simulink model "ejemplo_arduino"  (R2016a)
settings: Solver=ode3  StartTime=0.0  StopTime=inf  FixedStep=0.001  RelTol=1e-3
libraries: simulink x1, sldrtlib x1, aerolibanimutils x1
settings Model: Creator=Usuario  LastModifiedBy=santd
settings DataIOCC: LimitDataPoints=on  SaveFormat=Array
settings DebuggingCC: SolverPrmCheckMsg=warning  AllowSymbolicDim=off
settings HardwareCC: ProdBitPerPointer=32  ProdLargestAtomicFloat=None  ProdIntDivRoundTo=Undefined  ProdEndianess=Unspecified  ProdWordSize=32  ProdHWDeviceType=32-bit Generic
settings ModelReferenceCC: PropagateSignalLabelsOutOfModel=off
settings ConfigComp: CovModelRefEnable=Off  CovSFcnEnable=off

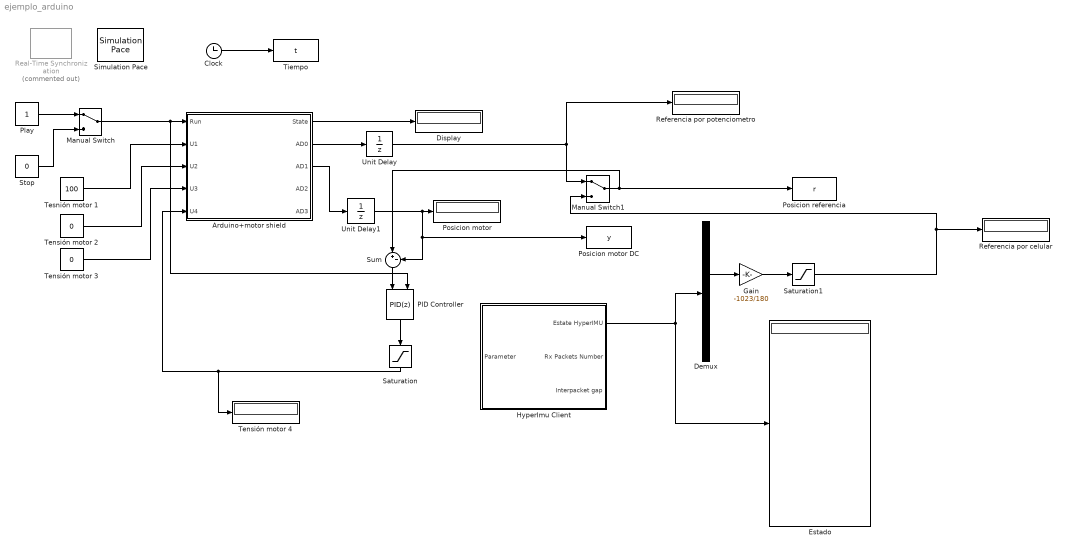
== system ejemplo_arduino ==
  Arduino+motor shield : Subsystem  mask{dev=1}
      mask prompts: dev "Device Number"
      mask Help:
      | HELP DEVICE
      | 
      | - App for using the kit arduino UNO plus Adafruit motor shield 1.2 based on two L293D chips forming 4 H-Bridges. L293D chipset provides 0.6A per bridge (1.2A peak) with thermal shutdown protection, internal kickback protection diodes. Can run motors on 4.5VDC to 25VDC. The shield is compatible with Arduino Mega 1280 & 2560, Diecimila, Duemilanove, and UNO
      | 
      | HELP DRIVERS
      | 
      | Upload the firmware 'Arduino_motor_firmware' in your Arduino UNO kit available from folder '\SAS TOOLS\Software arduino_motor V1.1.0'
      | -------------------------------------------------------------------------------------------------------------------------------------------------------
      | HELP APP
      | 
      | Before running the Simulink model initiate communication with the device through the application 'Arduino_motor.exe' available from folder '\SAS TOOLS\Software arduino_motor V1.1.0'. After executing the program the app icon is available in the taskbar.
      | The app "arduino_motor.exe" is handled from right-click on the icon and selecting the corresponding option:
      | "Play" -> Start the commnunication between the device and the app
      | "Stop" -> Stop the communication
      | "Monitor"->view the state of sensors and communication
      | 
      | -------------------------------------------------------------------------------------------------------------------------------------------------------
      | 
      | HELP BLOCK
      | 
      | Input Ports
      | 
      | Port 'Run': 1 for running and 0 for stopping
      | 
      | Port 'U1': value between [-255;255] which drives the tension applied to the motor 1 of the shield motor Adafruit 1.0
      | Port 'U2': value between [-255;255] which drives the tension applied to the motor 2 of the shield motor Adafruit 1.0
      | Port 'U3': value between [-255;255] which drives the tension applied to the motor 3 of the shield motor Adafruit 1.0
      | Port 'U4': value between [-255;255] which drives the tension applied to the motor 4 of the shield motor Adafruit 1.0
      | 
      | The range [-255;255] is related with the tension range [-V;V], where V is the tension source applied to the motor shield
      | 
      | Output Ports
      | 
      | Port 'State': information about the system. Run=1; Stop=0
      | 
      | Port 'AD0': value between [0;1023] measured in the pin AD0 of the Arduino UNO board
      | Port 'AD1': value between [0;1023] measured in the pin AD1 of the Arduino UNO board
      | Port 'AD2': value between [0;1023] measured in the pin AD2 of the Arduino UNO board
      | Port 'AD3': value between [0;1023] measured in the pin AD3 of the Arduino UNO board
      | 
      | The range [0;1023] is related with the tension range [0;5V] readed on the pins of the Arduino kit A/D conversor
      | -------------------------------------------------------------------------------------------------------------------------------------------------------
      | 
      | HELP SHARE MEMORY (information only for external applications different to "Arduino_motor.exe")
      | 
      | Shared Memory Names:
      | 
      | 'ARDUINO_entrada_'#dev
      | 'ARDUINO_salida_'#dev
      | NOTE: replace #dev with the device number
      mask DialogControl DescGroupVar Prompt: Arduino motor shield
      mask DialogControl DescTextVar Prompt: This block is used to receive and send data via USB port between a UNO Arduino board and the App "Arduino_motor.exe" available on folder '\SAS TOOLS\Software Arduino_motor V1.1.0'. You must upload the firmware "Arduino_motor_firmware" into your Arduino board. More information in Help button.
      mask Display:
      | image('motor_shield.png')
      | color('red')
      | port_label('input',1,'run')
      | port_label('input',2,'U1')
      | port_label('input',3,'U2')
      | port_label('input',4,'U3')
      | port_label('input',5,'U4')
      | color('blue')
      | port_label('output',1,'state')
      | port_label('output',2,'AD0')
      | port_label('output',3,'AD1')
      | port_label('output',4,'AD2')
      | port_label('output',5,'AD3')
  Clock : Clock
  Demux : Demux  Outputs=12
  Display : Display
  Estado : Display
  Gain : Gain  Gain=-1023/180
  HyperImu Client : Subsystem  mask{dev=2}
      mask prompts: dev "Device Number"
      mask Help:
      | HELP DEVICE
      | 
      | - UDP Client for the server "HyperIMU"-Android App
      | 
      | HELP DRIVERS
      | 
      | Install in your phone the app "HyperIMU" for Android. Link: https://play.google.com/store/apps/details?id=com.ianovir.hyper_imu&hl=es
      | -------------------------------------------------------------------------------------------------------------------------------------------------------
      | HELP APP
      | 
      | Before running the Simulink model initiate communication with the device through the application 'imu.exe' available from folder '\SAS TOOLS\Software imu V1.1.0'. After executing the program the app icon is available in the taskbar.
      | The app "HyperIMU.exe" is handled from right-click on the icon and selecting the corresponding option:
      | "Play" -> Start the commnunication between the device and the app
      | "Stop" -> Stop the communication
      | "Monitor"->view the state of sensors and communication
      | 
      | -------------------------------------------------------------------------------------------------------------------------------------------------------
      | 
      | HELP BLOCK
      | 
      | Input Ports
      | 
      | Port 'Parameters' scalar non-used.
      | 
      | Output Ports
      | 
      | Port 'State': sensors information chosen with the App HyperIMU
      | 
      | 'Rx Packets Number' number of received packets by the client
      | 
      | 'Interpacket gap' time between packets
      | 
      | -------------------------------------------------------------------------------------------------------------------------------------------------------
      | 
      | HELP SHARE MEMORY (information only for external applications different to "HyperIMU.exe")
      | 
      | Shared Memory Names:
      | 
      | 'HYPERIMU_entrada_'#dev
      | 'HYPERIMU_salida_'#dev
      | NOTE: replace #dev with the device number
      mask DialogControl DescGroupVar Prompt: HyperIMU client
      mask DialogControl DescTextVar Prompt: This block is used to receive data via UDP from the App "HyperIMU" through the application 'HyperIMU.exe' available on folder '\SAS TOOLS\Software HyperIMU V1.1.0'. More information in Help button.
      mask Display:
      | image('HyperIMU.png')
      | color('red')
      | port_label('input',1,'Parameter')
      | 
      | color('blue')
      | port_label('output',1,'State HyperIMU')
      | port_label('output',2,'Rx Packets Number')
      | port_label('output',3,'Interpacket gap')
  Manual Switch : ManualSwitch
  Manual Switch1 : ManualSwitch
  PID Controller : simulink/Continuous/PID Controller  Controller=PID  TimeDomain=Discrete-time  SampleTime=-1  IntegratorMethod=Forward Euler  FilterMethod=Forward Euler  Form=Parallel  UseFilter=on  ControllerParametersSource=internal  P=1.25  I=0.1  D=0.001  N=100  InitialConditionSource=internal  InitialConditionForIntegrator=0  InitialConditionForFilter=0  ExternalReset=either  ZeroCross=off  LimitOutput=on  UpperSaturationLimit=inf  LowerSaturationLimit=-inf  LinearizeAsGain=on  AntiWindupMode=back-calculation  Kb=1  TrackingMode=off  Kt=1  PParamMin=[]  PParamMax=[]  IParamMin=[]  IParamMax=[]  DParamMin=[]  DParamMax=[]  NParamMin=[]  NParamMax=[]  KbParamMin=[]  KbParamMax=[]  KtParamMin=[]  KtParamMax=[]  POutMin=[]  POutMax=[]  IOutMin=[]  IOutMax=[]  DOutMin=[]  DOutMax=[]  NOutMin=[]  NOutMax=[]  KbOutMin=[]  KbOutMax=[]  KtOutMin=[]  KtOutMax=[]  IntegratorOutMin=[]  IntegratorOutMax=[]  FilterOutMin=[]  FilterOutMax=[]  SumOutMin=[]  SumOutMax=[]  SumI1OutMin=[]  SumI1OutMax=[]  SumI2OutMin=[]  SumI2OutMax=[]  SumI3OutMin=[]  SumI3OutMax=[]  SumDOutMin=[]  SumDOutMax=[]  SaturationOutMin=[]  SaturationOutMax=[]  IntegratorContinuousStateAttributes=''  IntegratorStateMustResolveToSignalObject=off  IntegratorRTWStateStorageClass=Auto  FilterContinuousStateAttributes=''  FilterStateMustResolveToSignalObject=off  FilterRTWStateStorageClass=Auto  DifferentiatorICPrevScaledInput=0  DifferentiatorOutMin=[]  DifferentiatorOutMax=[]
  Play : Constant  OutDataTypeStr=single
  Posicion motor : Display
  Posicion motor DC : ToWorkspace  VariableName=y  SampleTime=-1
  Posicion referencia : ToWorkspace  VariableName=r  SampleTime=-1
  Real-Time Synchronization : sldrtlib/Real-Time Synchronization  Commented=on  SampleTime=0.001  MaxMissedTicks=inf  ShowMissedTicks=off  YieldWhenWaiting=off
  Referencia por celular : Display
  Referencia por potenciometro : Display
  Saturation : Saturate  UpperLimit=255  LowerLimit=-255  OutDataTypeStr=single
  Saturation1 : Saturate  UpperLimit=1023  LowerLimit=0  OutDataTypeStr=single
  Simulation Pace : aerolibanimutils/Simulation Pace  SimulationPace=1  SleepMode=MATLAB Thread  OutputPaceError=off  SampleTime=-1
  Stop : Constant  Value=0  OutDataTypeStr=single
  Sum : Sum  Inputs=|+-
  Tensión motor 2 : Constant  Value=0  OutDataTypeStr=single
  Tensión motor 3 : Constant  Value=0  OutDataTypeStr=single
  Tensión motor 4 : Display
  Tesnión motor 1 : Constant  Value=100  OutDataTypeStr=single
  Tiempo : ToWorkspace  VariableName=t  SampleTime=-1
  Unit Delay : UnitDelay  SampleTime=-1
  Unit Delay1 : UnitDelay  SampleTime=-1
  wires:
  Arduino+motor shield/1(State) -> Display/1
  Play/1 -> Manual Switch/1
  Stop/1 -> Manual Switch/2
  Manual Switch/1 -> PID Controller/2, Arduino+motor shield/1(Run)
  Clock/1 -> Tiempo/1
  Tesnión motor 1/1 -> Arduino+motor shield/2(U1)
  Tensión motor 2/1 -> Arduino+motor shield/3(U2)
  Tensión motor 3/1 -> Arduino+motor shield/4(U3)
  Sum/1 -> PID Controller/1
  PID Controller/1 -> Saturation/1
  Saturation/1 -> Tensión motor 4/1, Arduino+motor shield/5(U4)
  Unit Delay/1 -> Manual Switch1/1, Referencia por potenciometro/1
  Arduino+motor shield/2(AD0) -> Unit Delay/1
  Arduino+motor shield/3(AD1) -> Unit Delay1/1
  Unit Delay1/1 -> Posicion motor DC/1, Sum/2, Posicion motor/1
  HyperImu Client/1(Estate HyperIMU) -> Demux/1, Estado/1
  Manual Switch1/1 -> Posicion referencia/1, Sum/1
  Demux/5 -> Gain/1
  Gain/1 -> Saturation1/1
  Saturation1/1 -> Referencia por celular/1, Manual Switch1/2

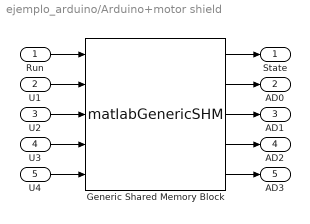
== system ejemplo_arduino/Arduino+motor shield ==
  Run : Inport
  U1 : Inport  Port=2
  U2 : Inport  Port=3
  U3 : Inport  Port=4
  U4 : Inport  Port=5
  Generic Shared Memory Block : S-Function  FunctionName=matlabGenericSHM  Parameters=nombre,dispositivo,vecE,vecS,tipoE,tipoS  SFunctionDeploymentMode=off  EnableBusSupport=off  mask(Generic Share Memory block V2.0){nombre='ARDUINO', dispositivo=dev, vecE=[1 1 1 1 1], vecS=[1 1 1 1 1], tipoE=['f' 'f' 'f' 'f' 'f'], tipoS=['f' 'f' 'f' 'f' 'f']}
      mask prompts: nombre "Share Memory base name"; dispositivo "Device Number"; vecE "Sizes input vector"; vecS "Sizes output vector"; tipoE "Data Types Inputs"; tipoS "Data Types Outputs"
      mask help:
      | This block allows Simulink communication with external processes through shared memory. It works on Unix and Windows.
      | More information in Help.
      mask Help:
      | Share Memory base name (nombre): It's the base string of share memory ej 'robot'
      | Device Number (dispositivo): integer that identifies the device between multiple in use
      | Two shared memorys are created with names:
      | "%name_entrada_%dispositivo" for the device input (writing)
      | "%name_salida_%dispositivo" for the device output (reading)
      | Sizes input vector (vecE)  : array that specify the number of inputs (array dimension) and the inputs size (array values)
      | Sizes output vector  (vecS): array that specify the number of outputs (array dimension) and the outputs size (array values)
      | Data types input(tipoE): char array that specify each input types
      | Data types output (tipoS): char array that specify each output types
      | Allowed types are:
      | ('f'=float, 'd'=double, 'i'=int32, 'c'=char, 'C'= unsigned char, 'I'=unsigned int)
      | Example.
      | Suppose the following parameters:
      | nombre='exampleMemory'
      | dispositivo=10
      | vecE=[3 2 1]
      | vecS=[6 5 7 8]
      | tipoE=['f' 'I' 'c']
      | tipoS=['C' 'i' 'd' 'd']
      | 
      | Two Share Memories are created with names:
      | "exampleMemory_entrada_10" (block input)
      | "exampleMemory_salida_10"  (block output)
      | 3 inputs are created:
      |  1° Dimension 3, type "unsigned char"
      |  2° Dimension 2, type "int"
      |  3° Dimension 1, type "char"
      | 4 outputs are created:
      |  1° Dimension 6, type "float"
      |  2° Dimension 5, type "unsigned int"
      |  3° Dimension 7, type "double"
      |  3° Dimension 8, type "double"
      mask Display: image('shmem.jpg')
  State : Outport
  AD0 : Outport  Port=2
  AD1 : Outport  Port=3
  AD2 : Outport  Port=4
  AD3 : Outport  Port=5
  wires:
  Generic Shared Memory Block/5 -> AD3/1
  Generic Shared Memory Block/4 -> AD2/1
  Generic Shared Memory Block/3 -> AD1/1
  Generic Shared Memory Block/2 -> AD0/1
  Generic Shared Memory Block/1 -> State/1
  U4/1 -> Generic Shared Memory Block/5
  U3/1 -> Generic Shared Memory Block/4
  U2/1 -> Generic Shared Memory Block/3
  U1/1 -> Generic Shared Memory Block/2
  Run/1 -> Generic Shared Memory Block/1

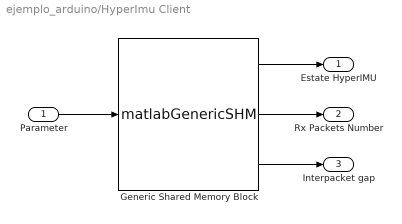
== system ejemplo_arduino/HyperImu Client ==
  Parameter : Inport
  Generic Shared Memory Block : S-Function  FunctionName=matlabGenericSHM  Parameters=nombre,dispositivo,vecE,vecS,tipoE,tipoS  SFunctionDeploymentMode=off  EnableBusSupport=off  mask(Generic Share Memory block V2.0){nombre='HYPERIMU', dispositivo=dev, vecE=[1], vecS=[12 1 1], tipoE=['f'], tipoS=['f' 'I' 'f']}
      mask prompts: nombre "Share Memory base name"; dispositivo "Device Number"; vecE "Sizes input vector"; vecS "Sizes output vector"; tipoE "Data Types Inputs"; tipoS "Data Types Outputs"
      mask help:
      | This block allows Simulink communication with external processes through shared memory. It works on Unix and Windows.
      | More information in Help.
      mask Help:
      | Share Memory base name (nombre): It's the base string of share memory ej 'robot'
      | Device Number (dispositivo): integer that identifies the device between multiple in use
      | Two shared memorys are created with names:
      | "%name_entrada_%dispositivo" for the device input (writing)
      | "%name_salida_%dispositivo" for the device output (reading)
      | Sizes input vector (vecE)  : array that specify the number of inputs (array dimension) and the inputs size (array values)
      | Sizes output vector  (vecS): array that specify the number of outputs (array dimension) and the outputs size (array values)
      | Data types input(tipoE): char array that specify each input types
      | Data types output (tipoS): char array that specify each output types
      | Allowed types are:
      | ('f'=float, 'd'=double, 'i'=int32, 'c'=char, 'C'= unsigned char, 'I'=unsigned int)
      | Example.
      | Suppose the following parameters:
      | nombre='exampleMemory'
      | dispositivo=10
      | vecE=[3 2 1]
      | vecS=[6 5 7 8]
      | tipoE=['f' 'I' 'c']
      | tipoS=['C' 'i' 'd' 'd']
      | 
      | Two Share Memories are created with names:
      | "exampleMemory_entrada_10" (block input)
      | "exampleMemory_salida_10"  (block output)
      | 3 inputs are created:
      |  1° Dimension 3, type "unsigned char"
      |  2° Dimension 2, type "int"
      |  3° Dimension 1, type "char"
      | 4 outputs are created:
      |  1° Dimension 6, type "float"
      |  2° Dimension 5, type "unsigned int"
      |  3° Dimension 7, type "double"
      |  3° Dimension 8, type "double"
      mask Display: image('shmem.jpg')
  Estate HyperIMU : Outport
  Rx Packets Number : Outport  Port=2
  Interpacket gap : Outport  Port=3
  wires:
  Generic Shared Memory Block/2 -> Rx Packets Number/1
  Generic Shared Memory Block/3 -> Interpacket gap/1
  Generic Shared Memory Block/1 -> Estate HyperIMU/1
  Parameter/1 -> Generic Shared Memory Block/1
